simulink model "蹦极"  (R2018b)
settings: Solver=VariableStepAuto  StartTime=0.0  StopTime=50  RelTol=1e-3
settings Model: Creator=Jason  LastModifiedBy=Jason

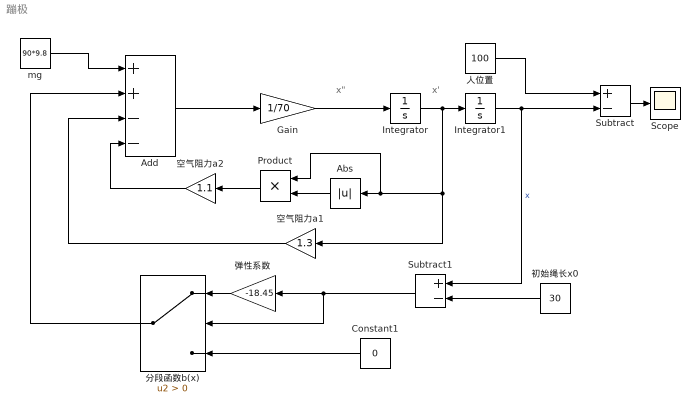
== system 蹦极 ==
  note: x'
  note: x"
  Abs : Abs
  Add : Sum  Inputs=++--
  Constant1 : Constant  Value=0
  Gain : Gain  Gain=1/70
  Integrator : Integrator
  Integrator1 : Integrator
  Product : Product
  Scope : Scope
  Subtract : Sum  Inputs=+-
  Subtract1 : Sum  Inputs=+-
  mg : Constant  Value=90*9.8
  人位置 : Constant  Value=100
  分段函数b(x) : Switch  Criteria=u2 > Threshold
  初始绳长x0 : Constant  Value=30
  弹性系数 : Gain  Gain=-18.45
  空气阻力a1 : Gain  Gain=1.3
  空气阻力a2 : Gain  Gain=1.1
  wires:
  mg/1 -> Add/1
  Add/1 -> Gain/1
  Gain/1 -> Integrator/1
  人位置/1 -> Subtract/1
  Subtract/1 -> Scope/1
  空气阻力a2/1 -> Add/4
  Product/1 -> 空气阻力a2/1
  Abs/1 -> Product/2
  空气阻力a1/1 -> Add/3
  Integrator1/1 -> Subtract1/1, Subtract/2  "x"
  弹性系数/1 -> 分段函数b(x)/1
  Constant1/1 -> 分段函数b(x)/3
  Subtract1/1 -> 弹性系数/1, 分段函数b(x)/2
  初始绳长x0/1 -> Subtract1/2
  Integrator/1 -> Product/1, Abs/1, 空气阻力a1/1, Integrator1/1
  分段函数b(x)/1 -> Add/2
